simulink model "hw01_Fig1b"  (R2024b)
settings: Solver=ode23tb  StartTime=0.0  StopTime=0.2  FixedStep=0.0001  MaxStep=0.01  RelTol=0.001  AbsTol=0.001
undefined symbols (not defined in the file): C_cap, L_1, L_2, r_C, r_L1, r_L2, r_leak
settings Model: Creator=Aryan Ritwajeet Jha  LastModifiedBy=aryan

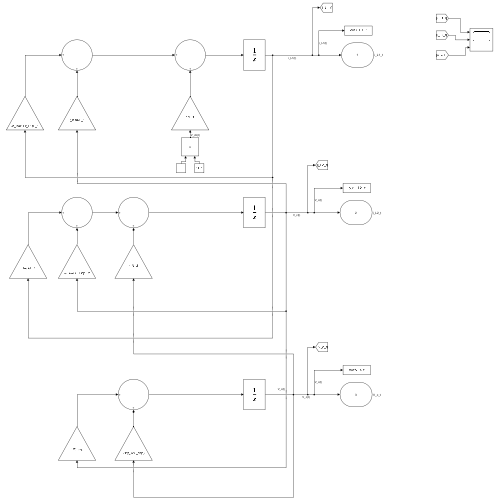
[thumbnail: Simulink's stored preview of the top-level diagram]
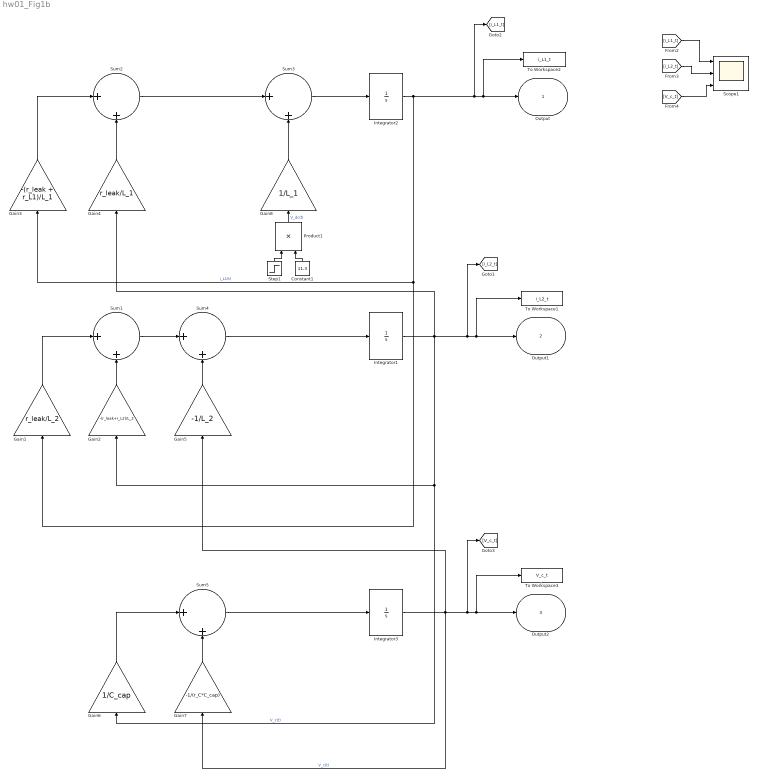
== system hw01_Fig1b ==
  Constant1 : Constant  Value=11.3
  Gain1 : Gain  Gain=r_leak/L_2
  Gain2 : Gain  Gain=-(r_leak+r_L2)/L_2
  Gain3 : Gain  Gain=-(r_leak + r_L1)/L_1
  Gain4 : Gain  Gain=r_leak/L_1
  Gain5 : Gain  Gain=-1/L_2
  Gain6 : Gain  Gain=1/C_cap
  Gain7 : Gain  Gain=-1/(r_C*C_cap)
  Gain8 : Gain  Gain=1/L_1
  Integrator1 : Integrator  ContinuousStateAttributes='i_L2_t'
  Integrator2 : Integrator  ContinuousStateAttributes='i_L1_t'
  Integrator3 : Integrator  ContinuousStateAttributes='V_c_t'
  Product1 : Product
  Scope1 : Scope  NumInputPorts=3
  Step1 : Step  Time=0  SampleTime=0
  Sum{1..5} (5 alike) : Sum  Inputs=|++
  To Workspace1 : ToWorkspace  VariableName=i_L2_t  SaveFormat=Timeseries  SampleTime=-1
  To Workspace2 : ToWorkspace  VariableName=i_L1_t  SaveFormat=Timeseries  SampleTime=-1
  To Workspace3 : ToWorkspace  VariableName=V_c_t  SaveFormat=Timeseries  SampleTime=-1
  Output : Outport  SignalName=i_L1_t
  Output1 : Outport  Port=2  SignalName=i_L2_t
  Output2 : Outport  Port=3  SignalName=V_c_t
  wires:
  Gain3/1 -> Sum2/1
  Gain4/1 -> Sum2/2
  Sum2/1 -> Sum3/1
  Step1/1 -> Product1/1
  Product1/1 -> Gain8/1  "V_dc(t)"
  Constant1/1 -> Product1/2
  Sum3/1 -> Integrator2/1
  [i_L1_t] -> Scope1/1
  [i_L2_t] -> Scope1/2
  Integrator2/1 -> Gain3/1, Gain1/1, [i_L1_t], To Workspace2/1, Output/1  "i_L1(t)"
  [V_c_t] -> Scope1/3
  Gain1/1 -> Sum1/1
  Sum1/1 -> Sum4/1
  Gain2/1 -> Sum1/2
  Gain5/1 -> Sum4/2
  Sum4/1 -> Integrator1/1
  Gain7/1 -> Sum5/2
  Integrator1/1 -> Gain6/1, Gain2/1, Gain4/1, [i_L2_t], To Workspace1/1, Output1/1  "V_c(t)"
  Gain6/1 -> Sum5/1
  Integrator3/1 -> Gain5/1, [V_c_t], To Workspace3/1, Output2/1, Gain7/1  "V_c(t)"
  Sum5/1 -> Integrator3/1
  Gain8/1 -> Sum3/2
